simulink model "VibrationAbsorber"  (R2020b)
settings: Solver=VariableStepAuto  StartTime=0.0  StopTime=10.0  MaxStep=0.002  RelTol=1e-3
values from neighbouring files (symbols this model uses):
  b = 50    [ToIntializePara.m]
  k1 = 50    [ToIntializePara.m]
  M1 = 100    [ToIntializePara.m]
settings Model: Creator=BIDITA PAUL  LastModifiedBy=BIDITA PAUL

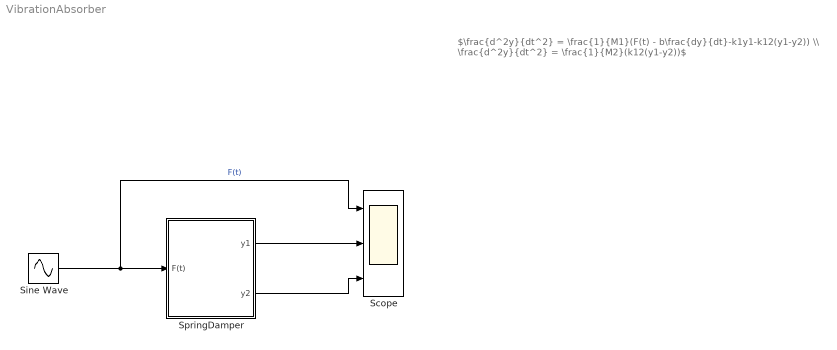
== system VibrationAbsorber ==
  note: $\frac{d^2y}{dt^2} = \frac{1}{M1}(F(t) - b\frac{dy}{dt}-k1y1-k12(y1-y2)) \\ \frac{d^2y}{dt^2} = \frac{1}{M2}(k12(y1-y2))$
  Scope : Scope  NumInputPorts=3
  Sine Wave : Sin  Amplitude=2  Frequency=10  SampleTime=0
  SpringDamper : Subsystem
  wires:
  Sine Wave/1 -> SpringDamper/1(F(t)), Scope/1  "F(t)"
  SpringDamper/1(y1) -> Scope/2
  SpringDamper/2(y2) -> Scope/3

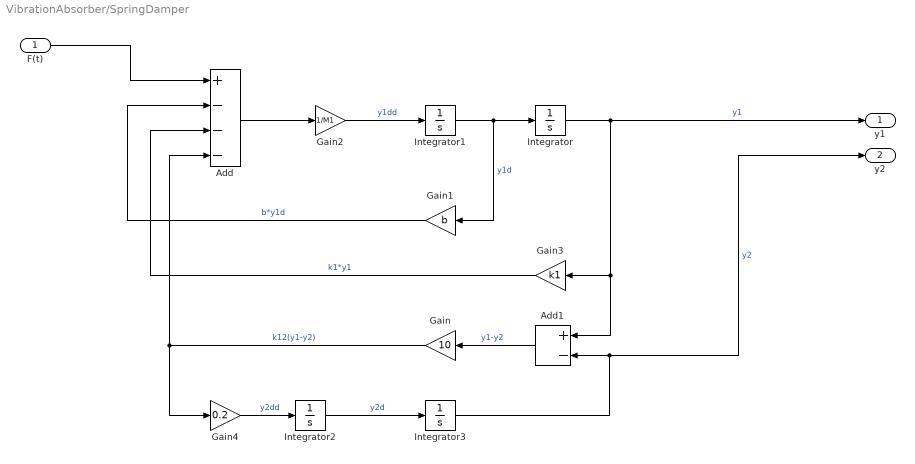
== system VibrationAbsorber/SpringDamper ==
  F(t) : Inport
  Add : Sum  Inputs=+---
  Add1 : Sum  Inputs=+-
  Gain : Gain  Gain=10
  Gain1 : Gain  Gain=b
  Gain2 : Gain  Gain=1/M1
  Gain3 : Gain  Gain=k1
  Gain4 : Gain  Gain=0.2
  Integrator{,1..3} (4 alike) : Integrator
  y1 : Outport
  y2 : Outport  Port=2
  wires:
  Gain2/1 -> Integrator1/1  "y1dd"
  Gain1/1 -> Add/2  "b*y1d"
  Integrator3/1 -> y2/1, Add1/2  "y2"
  Integrator1/1 -> Gain1/1, Integrator/1  "y1d"
  Gain/1 -> Gain4/1, Add/4  "k12(y1-y2)"
  Add1/1 -> Gain/1  "y1-y2"
  Integrator/1 -> y1/1, Add1/1, Gain3/1  "y1"
  Integrator2/1 -> Integrator3/1  "y2d"
  F(t)/1 -> Add/1
  Gain3/1 -> Add/3  "k1*y1"
  Gain4/1 -> Integrator2/1  "y2dd"
  Add/1 -> Gain2/1
